simulink library "rocket_thrust_curve_library"  (R2014a)
settings: Solver=ode45  StartTime=0.0  StopTime=10.0  RelTol=1e-3
settings Model: Creator=scorpii  LastModifiedBy=scorpii

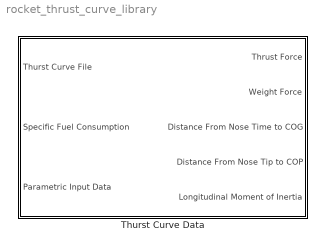
== system rocket_thrust_curve_library ==
  Thurst Curve Data : Subsystem

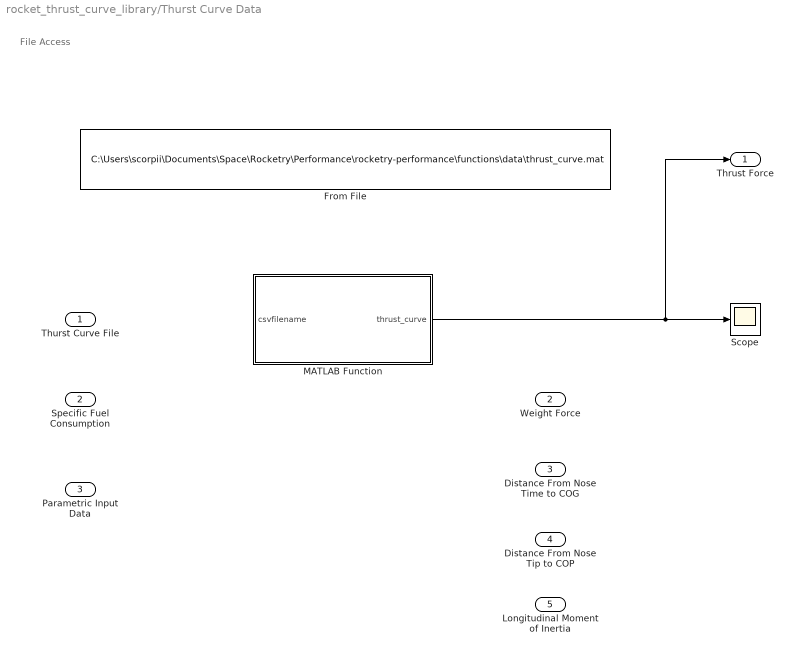
== system rocket_thrust_curve_library/Thurst Curve Data ==
  note: File Access
  Thurst Curve File : Inport
  "Specific Fuel Consumption " : Inport  Port=2
  Parametric Input Data : Inport  Port=3
  From File : FromFile  FileName=C:\Users\scorpii\Documents\Space\Rocketry\Performance\rocketry-performance\functions\data\thrust_curve.mat  SampleTime=0.01
  MATLAB Function : MATLAB Function  TreatAsAtomicUnit=on
  Scope : Scope
  Thrust Force : Outport
  Weight Force : Outport  Port=2
  Distance From Nose Time to COG : Outport  Port=3
  Distance From Nose Tip to COP : Outport  Port=4
  Longitudinal Moment of Inertia : Outport  Port=5
  wires:
  MATLAB Function/1(thrust_curve) -> Scope/1, Thrust Force/1

== matlab function rocket_thrust_curve_library/Thurst Curve Data/MATLAB Function ==
  data: csvfilename input; thrust_curve output
function thrust_curve = thrust_data_import_temp(csvfilename)
%-------------------------------------------------------------------------------
%
% thrust_data_import.m
%
% Data Access of Parametric Model
%
% Thrust curves are provided in tabulated and time-based form. The values for 
% thrust need to be processed as input to the model in a synchronized fashion
% with the simulation clock
%
% A csvfilename shall be provided for a CSV file containing in the first column
% the time and in the secoond column the thrust force
%
% The data is read using xlsread and transposed for a lookup table to change
% the data
% 
% TODO The data should be interpolated to keep the time-step constant
% 
% Important Notes:
% Time values need to be monotomically non-decreasing. Meaning, the time
% step must be equal or increasing only. As such, the smallest time-step
% should be chosen and the data in between interpolated to complete the 
% set. TODO
%
%-------------------------------------------------------------------------------
% References
% http://www.mathworks.com/help/simulink/ug/how-to-import-data-from-an-excel-spreadsheet.html
% http://www.mathworks.com/help/matlab/matlab_external/example-reading-excel-spreadsheet-data.html
%-------------------------------------------------------------------------------

% Import the data from Excel
% data = xlsread(csvfilename);

% TODO hardcoding is bad
data = xlsread('monotomic_time_thrust_curve.csv');

% Interpolate the data
% data = scrd_interpolate(data)

% Transpose the data for the .mat file
data_transpose = data.';

% Store the data in a .mat file
save('thrust_curve.mat','data_transpose');

% Extract data from mat file
time = data(:,1);
thrust = data(:,2);

% Plot the thrust curve for reference
% TODO: maybe we want to ask the user to verify the curve before proceeding
%plot(time,thrust);

thrust_curve = data_transpose;

% Row indices for lookup table
% breakpoints1 = data(2:end,1)';

% Column indices for lookup table
% breakpoints2 = data(1,2:end);

% output values for lookup table
% table_data = data(2:end,2:end);
